simulink model "controlador_on_off"  (R2015a)
settings: Solver=ode45  StartTime=0.0  StopTime=10.0  RelTol=1e-3
values from neighbouring files (symbols this model uses):
  C1 = 200    [controlador_on_off.m]
  C2 = -200    [controlador_on_off.m]
libraries: cstblocks x2
settings Model: Creator=Jose Roldan  LastModifiedBy=Jose Roldan

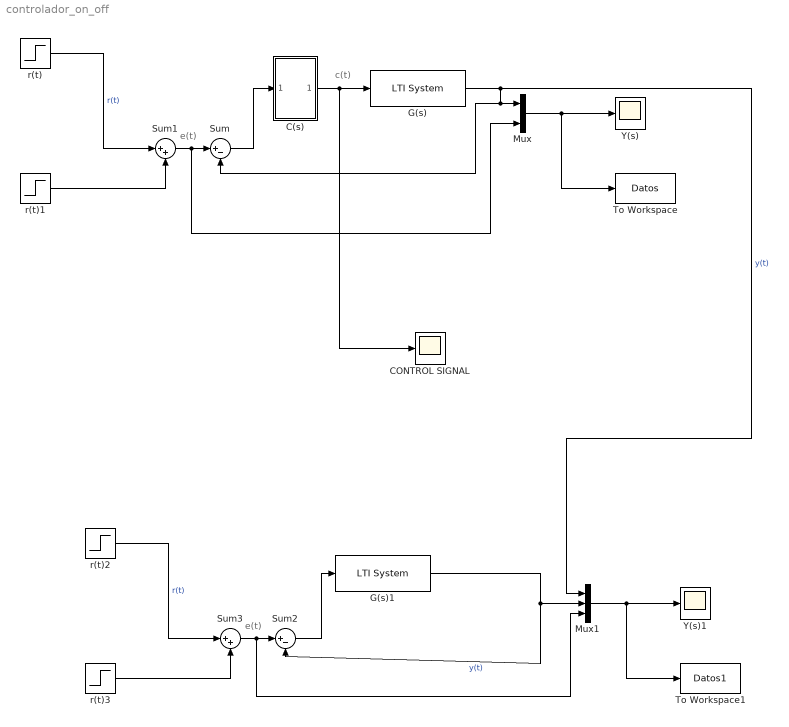
== system controlador_on_off ==
  note: c(t)
  note: e(t)
  note: e(t)
  C(s) : Subsystem
  CONTROL SIGNAL : Scope
  G(s) : cstblocks/LTI System  sys=G  IC=[]
  G(s)1 : cstblocks/LTI System  sys=G  IC=[]
  Mux : Mux  Inputs=2
  Mux1 : Mux  Inputs=3
  Sum : Sum  Inputs=|+-
  Sum1 : Sum  Inputs=|++
  Sum2 : Sum  Inputs=|+-
  Sum3 : Sum  Inputs=|++
  To Workspace : ToWorkspace  VariableName=Datos  SaveFormat=Structure With Time  SampleTime=-1
  To Workspace1 : ToWorkspace  VariableName=Datos1  SaveFormat=Structure With Time  SampleTime=-1
  Y(s) : Scope
  Y(s)1 : Scope
      settings: SaveName=ScopeData3
  r(t) : Step  Time=0  Before=5  After=10  SampleTime=0
  r(t)1 : Step  Time=5  Before=10  After=40  SampleTime=0
  r(t)2 : Step  Time=0  Before=5  After=10  SampleTime=0
  r(t)3 : Step  Time=5  Before=10  After=40  SampleTime=0
  wires:
  r(t)/1 -> Sum1/1  "r(t)"
  r(t)1/1 -> Sum1/2
  G(s)/1 -> Mux1/1, Sum/2, Mux/1  "y(t)"
  Mux/1 -> Y(s)/1, To Workspace/1
  C(s)/1(y(t)) -> CONTROL SIGNAL/1, G(s)/1
  Sum1/1 -> Mux/2, Sum/1
  Sum/1 -> C(s)/1(e(t))
  r(t)2/1 -> Sum3/1  "r(t)"
  r(t)3/1 -> Sum3/2
  G(s)1/1 -> Mux1/2, Sum2/2  "y(t)"
  Mux1/1 -> Y(s)1/1, To Workspace1/1
  Sum3/1 -> Mux1/3, Sum2/1
  Sum2/1 -> G(s)1/1

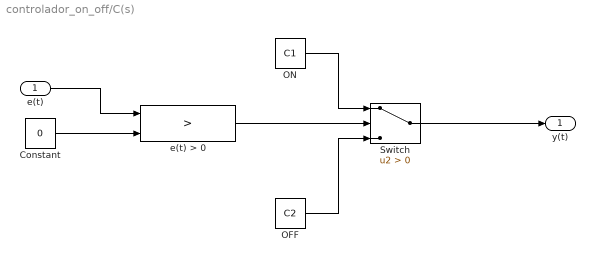
== system controlador_on_off/C(s) ==
  e(t) : Inport
  Constant : Constant  Value=0
  OFF : Constant  Value=C2
  "ON " : Constant  Value=C1
  Switch : Switch  Criteria=u2 > Threshold
  e(t) > 0 : RelationalOperator  Operator=>  OutDataTypeStr=boolean  ZeroCross=off
  y(t) : Outport
  wires:
  "ON "/1 -> Switch/1
  e(t) > 0/1 -> Switch/2
  OFF/1 -> Switch/3
  e(t)/1 -> e(t) > 0/1
  Switch/1 -> y(t)/1
  Constant/1 -> e(t) > 0/2
